simulink model "Orzan_Catalin_Matlab_Simulink"  (R2016a)
settings: Solver=VariableStepAuto  StartTime=0.0  StopTime=10.0  RelTol=1e-3
libraries: mblibv1 x17, simulink_extras x5
settings Model: Creator=Cata  LastModifiedBy=Cata

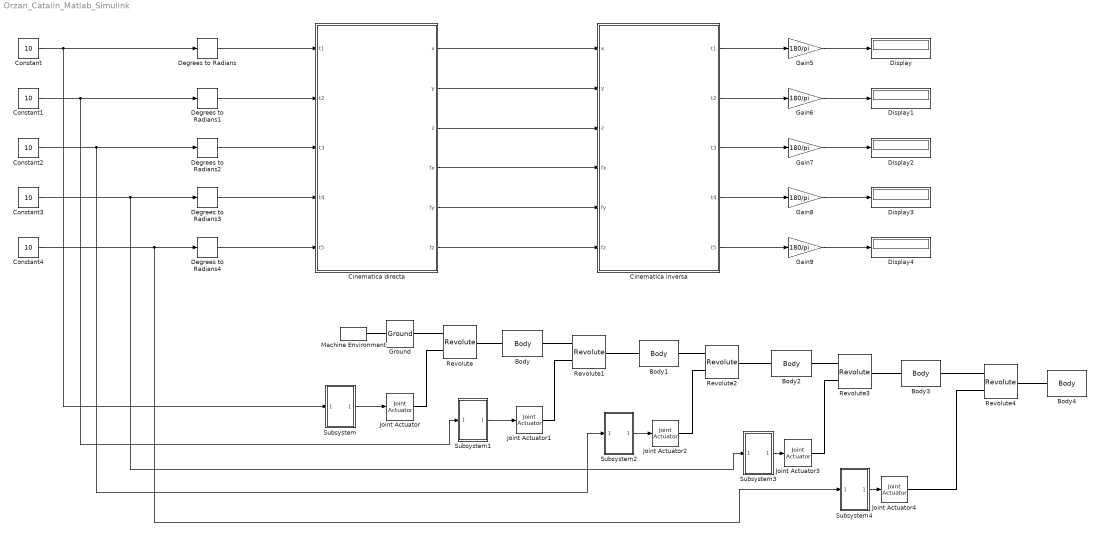
== system Orzan_Catalin_Matlab_Simulink ==
  Body : mblibv1/Bodies/Body  LConnTagsString=CS1  RConnTagsString=CS2  UpdateFromCAD=off  DialogClass=MechanicalBodyBlock  Mass=1  MassUnits=kg  InertiaUnits=kg*m^2  Inertia=eye(3)  Shape=Cylinder  ShapeDims=[1 1]  ShapeUnits=m  ShapeUse=false  Density=1  DensityUnits=kg/m^3  DensityUse=false  GraphicsMode=MACHINE_DEFAULT  BodyColorSelMode=MACHINE_DEFAULT  BodyColor=[1 0 0]  AttachedToCS=CG  CG=Left$CG$[0 0 0]$WORLD$WORLD$mm$[0 0 0]$Euler X-Y-Z$deg$WORLD$false$none  WorkingFrames=Left$CS1$[0 0 0]$World$World$mm$[0 0 0]$Euler X-Y-Z$deg$WORLD$true$none#Right$CS2$[0 0 200]$World$World$mm$[0 0 0]$Euler X-Y-Z$deg$WORLD$true$none  CGPos=[0 0 0]  CGRot=[0 0 0]  CS0Pos=[]  CS0Rot=[]  CS1Pos=[0 0 0]  CS1Rot=[0 0 0]  CS2Pos=[0 0 200]  CS2Rot=[0 0 0]  CS3Pos=[]  CS3Rot=[]  CS4Pos=[]  CS4Rot=[]  CS5Pos=[]  CS5Rot=[]  CS6Pos=[]  CS6Rot=[]  CS7Pos=[]  CS7Rot=[]  CS8Pos=[]  CS8Rot=[]  CS9Pos=[]  CS9Rot=[]  CS10Pos=[]  CS10Rot=[]  CS11Pos=[]  CS11Rot=[]  CS12Pos=[]  CS12Rot=[]  CS13Pos=[]  CS13Rot=[]  CS14Pos=[]  CS14Rot=[]  CS15Pos=[]  CS15Rot=[]  CS16Pos=[]  CS16Rot=[]  CS17Pos=[]  CS17Rot=[]  CS18Pos=[]  CS18Rot=[]  CS19Pos=[]  CS19Rot=[]  CS20Pos=[]  CS20Rot=[]
  Body1 : mblibv1/Bodies/Body  LConnTagsString=CS1  RConnTagsString=CS2  UpdateFromCAD=off  DialogClass=MechanicalBodyBlock  Mass=1  MassUnits=kg  InertiaUnits=kg*m^2  Inertia=eye(3)  Shape=Cylinder  ShapeDims=[1 1]  ShapeUnits=m  ShapeUse=false  Density=1  DensityUnits=kg/m^3  DensityUse=false  GraphicsMode=MACHINE_DEFAULT  BodyColorSelMode=MACHINE_DEFAULT  BodyColor=[1 0 0]  AttachedToCS=CG  CG=Left$CG$[0 0 200]$WORLD$WORLD$mm$[0 0 0]$Euler X-Y-Z$deg$WORLD$false$none  WorkingFrames=Left$CS1$[0 0 200]$World$World$mm$[0 0 0]$Euler X-Y-Z$deg$WORLD$true$none#Right$CS2$[0 0 400]$World$World$mm$[0 0 0]$Euler X-Y-Z$deg$WORLD$true$none  CGPos=[0 0 200]  CGRot=[0 0 0]  CS0Pos=[]  CS0Rot=[]  CS1Pos=[0 0 200]  CS1Rot=[0 0 0]  CS2Pos=[0 0 400]  CS2Rot=[0 0 0]  CS3Pos=[]  CS3Rot=[]  CS4Pos=[]  CS4Rot=[]  CS5Pos=[]  CS5Rot=[]  CS6Pos=[]  CS6Rot=[]  CS7Pos=[]  CS7Rot=[]  CS8Pos=[]  CS8Rot=[]  CS9Pos=[]  CS9Rot=[]  CS10Pos=[]  CS10Rot=[]  CS11Pos=[]  CS11Rot=[]  CS12Pos=[]  CS12Rot=[]  CS13Pos=[]  CS13Rot=[]  CS14Pos=[]  CS14Rot=[]  CS15Pos=[]  CS15Rot=[]  CS16Pos=[]  CS16Rot=[]  CS17Pos=[]  CS17Rot=[]  CS18Pos=[]  CS18Rot=[]  CS19Pos=[]  CS19Rot=[]  CS20Pos=[]  CS20Rot=[]
  Body2 : mblibv1/Bodies/Body  LConnTagsString=CS1  RConnTagsString=CS2  UpdateFromCAD=off  DialogClass=MechanicalBodyBlock  Mass=1  MassUnits=kg  InertiaUnits=kg*m^2  Inertia=eye(3)  Shape=Cylinder  ShapeDims=[1 1]  ShapeUnits=m  ShapeUse=false  Density=1  DensityUnits=kg/m^3  DensityUse=false  GraphicsMode=MACHINE_DEFAULT  BodyColorSelMode=MACHINE_DEFAULT  BodyColor=[1 0 0]  AttachedToCS=CG  CG=Left$CG$[0 0 400]$WORLD$WORLD$mm$[0 0 0]$Euler X-Y-Z$deg$WORLD$false$none  WorkingFrames=Left$CS1$[0 0 400]$World$World$mm$[0 0 0]$Euler X-Y-Z$deg$WORLD$true$none#Right$CS2$[200 0 400]$World$World$mm$[0 0 0]$Euler X-Y-Z$deg$WORLD$true$none  CGPos=[0 0 400]  CGRot=[0 0 0]  CS0Pos=[]  CS0Rot=[]  CS1Pos=[0 0 400]  CS1Rot=[0 0 0]  CS2Pos=[200 0 400]  CS2Rot=[0 0 0]  CS3Pos=[]  CS3Rot=[]  CS4Pos=[]  CS4Rot=[]  CS5Pos=[]  CS5Rot=[]  CS6Pos=[]  CS6Rot=[]  CS7Pos=[]  CS7Rot=[]  CS8Pos=[]  CS8Rot=[]  CS9Pos=[]  CS9Rot=[]  CS10Pos=[]  CS10Rot=[]  CS11Pos=[]  CS11Rot=[]  CS12Pos=[]  CS12Rot=[]  CS13Pos=[]  CS13Rot=[]  CS14Pos=[]  CS14Rot=[]  CS15Pos=[]  CS15Rot=[]  CS16Pos=[]  CS16Rot=[]  CS17Pos=[]  CS17Rot=[]  CS18Pos=[]  CS18Rot=[]  CS19Pos=[]  CS19Rot=[]  CS20Pos=[]  CS20Rot=[]
  Body3 : mblibv1/Bodies/Body  LConnTagsString=CS1  RConnTagsString=CS2  UpdateFromCAD=off  DialogClass=MechanicalBodyBlock  Mass=10  MassUnits=kg  InertiaUnits=kg*m^2  Inertia=eye(3)  Shape=Cylinder  ShapeDims=[1 1]  ShapeUnits=m  ShapeUse=false  Density=1  DensityUnits=kg/m^3  DensityUse=false  GraphicsMode=MACHINE_DEFAULT  BodyColorSelMode=MACHINE_DEFAULT  BodyColor=[1 0 0]  AttachedToCS=CG  CG=Left$CG$[200 0 400]$WORLD$WORLD$mm$[0 0 0]$Euler X-Y-Z$deg$WORLD$false$none  WorkingFrames=Left$CS1$[200 0 400]$World$World$mm$[0 0 0]$Euler X-Y-Z$deg$WORLD$true$none#Right$CS2$[200 0 200]$World$World$mm$[0 0 0]$Euler X-Y-Z$deg$WORLD$true$none  CGPos=[200 0 400]  CGRot=[0 0 0]  CS0Pos=[]  CS0Rot=[]  CS1Pos=[200 0 400]  CS1Rot=[0 0 0]  CS2Pos=[200 0 200]  CS2Rot=[0 0 0]  CS3Pos=[]  CS3Rot=[]  CS4Pos=[]  CS4Rot=[]  CS5Pos=[]  CS5Rot=[]  CS6Pos=[]  CS6Rot=[]  CS7Pos=[]  CS7Rot=[]  CS8Pos=[]  CS8Rot=[]  CS9Pos=[]  CS9Rot=[]  CS10Pos=[]  CS10Rot=[]  CS11Pos=[]  CS11Rot=[]  CS12Pos=[]  CS12Rot=[]  CS13Pos=[]  CS13Rot=[]  CS14Pos=[]  CS14Rot=[]  CS15Pos=[]  CS15Rot=[]  CS16Pos=[]  CS16Rot=[]  CS17Pos=[]  CS17Rot=[]  CS18Pos=[]  CS18Rot=[]  CS19Pos=[]  CS19Rot=[]  CS20Pos=[]  CS20Rot=[]
  Body4 : mblibv1/Bodies/Body  LConnTagsString=CS1  UpdateFromCAD=off  DialogClass=MechanicalBodyBlock  Mass=10  MassUnits=kg  InertiaUnits=kg*m^2  Inertia=eye(3)  Shape=Cylinder  ShapeDims=[1 1]  ShapeUnits=m  ShapeUse=false  Density=1  DensityUnits=kg/m^3  DensityUse=false  GraphicsMode=MACHINE_DEFAULT  BodyColorSelMode=MACHINE_DEFAULT  BodyColor=[1 0 0]  AttachedToCS=CG  CG=Left$CG$[200 0 200]$WORLD$WORLD$mm$[0 0 0]$Euler X-Y-Z$deg$WORLD$false$none  WorkingFrames=Left$CS1$[200 0 200]$World$World$mm$[0 0 0]$Euler X-Y-Z$deg$WORLD$true$none#Right$CS2$[200 0 0]$World$World$mm$[0 0 0]$Euler X-Y-Z$deg$WORLD$false$none  CGPos=[200 0 200]  CGRot=[0 0 0]  CS0Pos=[]  CS0Rot=[]  CS1Pos=[200 0 200]  CS1Rot=[0 0 0]  CS2Pos=[200 0 0]  CS2Rot=[0 0 0]  CS3Pos=[]  CS3Rot=[]  CS4Pos=[]  CS4Rot=[]  CS5Pos=[]  CS5Rot=[]  CS6Pos=[]  CS6Rot=[]  CS7Pos=[]  CS7Rot=[]  CS8Pos=[]  CS8Rot=[]  CS9Pos=[]  CS9Rot=[]  CS10Pos=[]  CS10Rot=[]  CS11Pos=[]  CS11Rot=[]  CS12Pos=[]  CS12Rot=[]  CS13Pos=[]  CS13Rot=[]  CS14Pos=[]  CS14Rot=[]  CS15Pos=[]  CS15Rot=[]  CS16Pos=[]  CS16Rot=[]  CS17Pos=[]  CS17Rot=[]  CS18Pos=[]  CS18Rot=[]  CS19Pos=[]  CS19Rot=[]  CS20Pos=[]  CS20Rot=[]
  "Cinematica directa " : MATLAB Function  TreatAsAtomicUnit=on
  Cinematica inversa : MATLAB Function  TreatAsAtomicUnit=on
  Constant{,1..4} (5 alike) : Constant  Value=10
  Degrees to Radians{,1..4} (5 alike) : simulink_extras/Transformations/Degrees to Radians
  Display{,1..4} (5 alike) : Display
  Gain{5..9} (5 alike) : Gain  Gain=180/pi
  Ground : mblibv1/Bodies/Ground  UpdateFromCAD=off  LeftPortType=env  RightPortType=workingframe  PhysicalDomain=Mechanical  DialogClass=GroundBlock  CoordPosition=[0 0 0]  CoordPositionUnits=m  StateVectorMgrId=0  MachineId=[1 0]  ShowEnvPort=on  ParameterChecksum=[4168860495, 2563258822, 2023213708, 520383932]  TopologyChecksum=[1341745960, 1067854235, 1921025474, 1139980135]
  Joint Actuator{,1..4} (5 alike) : mblibv1/Sensors &  Actuators/Joint Actuator  UpdateFromCAD=off  PhysicalDomain=Mechanical  PortType=blob  ActuationStyle=Motion  AngleUnits=deg  ArcVelocityUnits=deg/s  ArcAccelerationUnits=deg/s^2  CoordPositionUnits=m  VelocityUnits=m/s  AccelerationUnits=m/s^2  ForceUnits=N  TorqueUnits=N*m  ActiveIO=on  Width=3  DialogClass=MechanicalActuatorBlock  Primitive=R1  ReferenceFrame=Absolute (World)
  Machine Environment : mblibv1/Bodies/Machine Environment  PortType=env  PhysicalDomain=Mechanical  DialogTemplateClass=MECH.MachineEnvironment  SyncWhenCopied=off  Gravity=[0 -9.81 0]  GravityUnits=m/s^2  GravityAsSignal=off  Dimensionality=Auto-detect  AnalysisType=Forward dynamics  LinearAssemblyTolerance=1e-3  LinearAssemblyToleranceUnits=m  AngularAssemblyTolerance=1e-3  AngularAssemblyToleranceUnits=rad  ConstraintSolverType=Stabilizing  ConstraintRelTolerance=1e-4  ConstraintAbsTolerance=1e-4  UseRobustSingularityHandling=off  RedundancyAnalysisToleranceType=Automatically select tolerance  RedundancyAnalysisTolerance=1e-14  StatePerturbationType=Fixed  PerturbationSize=1e-5  VisualizeMachine=on  BodyVisualizationType=Use model default body geometries  BodyColorSelMode=Use model default  DefaultBodyColor=[1 0 0]
  Revolute : mblibv1/Joints/Revolute  LConnTagsString=__newl0|SA1  RConnTagsString=__newr0  UpdateFromCAD=off  NumSAPorts=1  CutJoint=off  MarkAsCut=off  Primitives=prismatic  PrimitiveProps=R1$World$[0 0 1]$revolute  DialogClass=JointBlock  R1Axis=[0 0 1]
  Revolute1 : mblibv1/Joints/Revolute  LConnTagsString=__newl0|SA1  RConnTagsString=__newr0  UpdateFromCAD=off  NumSAPorts=1  CutJoint=off  MarkAsCut=off  Primitives=prismatic  PrimitiveProps=R1$World$[0 1 0]$revolute  DialogClass=JointBlock  R1Axis=[0 1 0]
  Revolute2 : mblibv1/Joints/Revolute  LConnTagsString=__newl0|SA1  RConnTagsString=__newr0  UpdateFromCAD=off  NumSAPorts=1  CutJoint=off  MarkAsCut=off  Primitives=prismatic  PrimitiveProps=R1$World$[0 1 0]$revolute  DialogClass=JointBlock  R1Axis=[0 1 0]
  Revolute3 : mblibv1/Joints/Revolute  LConnTagsString=__newl0|SA1  RConnTagsString=__newr0  UpdateFromCAD=off  NumSAPorts=1  CutJoint=off  MarkAsCut=off  Primitives=prismatic  PrimitiveProps=R1$World$[0 1 0]$revolute  DialogClass=JointBlock  R1Axis=[0 1 0]
  Revolute4 : mblibv1/Joints/Revolute  LConnTagsString=__newl0|SA1  RConnTagsString=__newr0  UpdateFromCAD=off  NumSAPorts=1  CutJoint=off  MarkAsCut=off  Primitives=prismatic  PrimitiveProps=R1$World$[1 0 0]$revolute  DialogClass=JointBlock  R1Axis=[1 0 0]
  Subsystem : Subsystem
  Subsystem1 : Subsystem
  Subsystem2 : Subsystem
  Subsystem3 : Subsystem
  Subsystem4 : Subsystem
  wires:
  Constant3/1 -> Subsystem3/1(In1), Degrees to Radians3/1
  Constant2/1 -> Subsystem2/1(In1), Degrees to Radians2/1
  Constant1/1 -> Subsystem1/1(In1), Degrees to Radians1/1
  Constant/1 -> Subsystem/1(In1), Degrees to Radians/1
  Subsystem/1(Out1) -> Joint Actuator/1
  Subsystem1/1(Out1) -> Joint Actuator1/1
  Subsystem2/1(Out1) -> Joint Actuator2/1
  Subsystem3/1(Out1) -> Joint Actuator3/1
  Subsystem4/1(Out1) -> Joint Actuator4/1
  Constant4/1 -> Subsystem4/1(In1), Degrees to Radians4/1
  Cinematica inversa/1(t1) -> Gain5/1
  Cinematica inversa/5(t5) -> Gain9/1
  Cinematica inversa/4(t4) -> Gain8/1
  Cinematica inversa/3(t3) -> Gain7/1
  Cinematica inversa/2(t2) -> Gain6/1
  Gain5/1 -> Display/1
  Gain9/1 -> Display4/1
  Gain8/1 -> Display3/1
  Gain7/1 -> Display2/1
  Gain6/1 -> Display1/1
  "Cinematica directa "/6(fz) -> Cinematica inversa/6(fz)
  "Cinematica directa "/5(fy) -> Cinematica inversa/5(fy)
  "Cinematica directa "/4(fx) -> Cinematica inversa/4(fx)
  "Cinematica directa "/3(z) -> Cinematica inversa/3(z)
  "Cinematica directa "/2(y) -> Cinematica inversa/2(y)
  "Cinematica directa "/1(x) -> Cinematica inversa/1(x)
  Degrees to Radians4/1 -> "Cinematica directa "/5(t5)
  Degrees to Radians3/1 -> "Cinematica directa "/4(t4)
  Degrees to Radians2/1 -> "Cinematica directa "/3(t3)
  Degrees to Radians1/1 -> "Cinematica directa "/2(t2)
  Degrees to Radians/1 -> "Cinematica directa "/1(t1)
  connections:
  Ground/RConn1 -- Revolute/LConn1
  Revolute/RConn1 -- Body/LConn1
  Body/RConn1 -- Revolute1/LConn1
  Revolute1/RConn1 -- Body1/LConn1
  Body1/RConn1 -- Revolute2/LConn1
  Revolute2/RConn1 -- Body2/LConn1
  Body2/RConn1 -- Revolute3/LConn1
  Revolute3/RConn1 -- Body3/LConn1
  Joint Actuator/RConn1 -- Revolute/LConn2
  Joint Actuator1/RConn1 -- Revolute1/LConn2
  Joint Actuator2/RConn1 -- Revolute2/LConn2
  Joint Actuator3/RConn1 -- Revolute3/LConn2
  Machine Environment/RConn1 -- Ground/LConn1
  Revolute4/RConn1 -- Body4/LConn1
  Revolute4/LConn1 -- Body3/RConn1
  Revolute4/LConn2 -- Joint Actuator4/RConn1

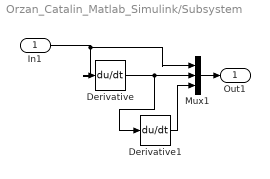
== system Orzan_Catalin_Matlab_Simulink/Subsystem ==
  In1 : Inport
  Derivative : Derivative
  Derivative1 : Derivative
  Mux1 : Mux  Inputs=3
  Out1 : Outport
  wires:
  Derivative/1 -> Derivative1/1, Mux1/2
  Mux1/1 -> Out1/1
  In1/1 -> Derivative/1, Mux1/1
  Derivative1/1 -> Mux1/3

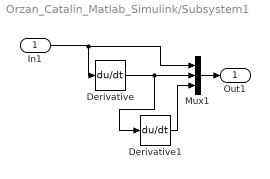
== system Orzan_Catalin_Matlab_Simulink/Subsystem1 ==
  In1 : Inport
  Derivative : Derivative
  Derivative1 : Derivative
  Mux1 : Mux  Inputs=3
  Out1 : Outport
  wires:
  Derivative/1 -> Derivative1/1, Mux1/2
  Mux1/1 -> Out1/1
  In1/1 -> Derivative/1, Mux1/1
  Derivative1/1 -> Mux1/3

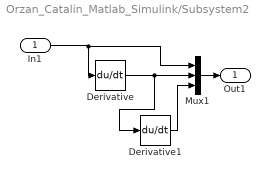
== system Orzan_Catalin_Matlab_Simulink/Subsystem2 ==
  In1 : Inport
  Derivative : Derivative
  Derivative1 : Derivative
  Mux1 : Mux  Inputs=3
  Out1 : Outport
  wires:
  Derivative/1 -> Derivative1/1, Mux1/2
  Mux1/1 -> Out1/1
  In1/1 -> Derivative/1, Mux1/1
  Derivative1/1 -> Mux1/3

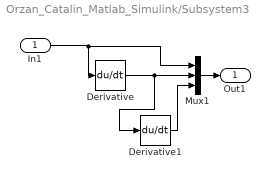
== system Orzan_Catalin_Matlab_Simulink/Subsystem3 ==
  In1 : Inport
  Derivative : Derivative
  Derivative1 : Derivative
  Mux1 : Mux  Inputs=3
  Out1 : Outport
  wires:
  Derivative/1 -> Derivative1/1, Mux1/2
  Mux1/1 -> Out1/1
  In1/1 -> Derivative/1, Mux1/1
  Derivative1/1 -> Mux1/3

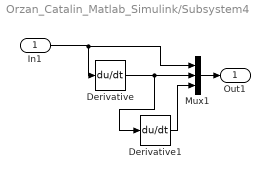
== system Orzan_Catalin_Matlab_Simulink/Subsystem4 ==
  In1 : Inport
  Derivative : Derivative
  Derivative1 : Derivative
  Mux1 : Mux  Inputs=3
  Out1 : Outport
  wires:
  Derivative/1 -> Derivative1/1, Mux1/2
  Mux1/1 -> Out1/1
  In1/1 -> Derivative/1, Mux1/1
  Derivative1/1 -> Mux1/3

== matlab function Orzan_Catalin_Matlab_Simulink/Cinematica inversa ==
  data: t1 output; x input; t2 output; y input; z input; fx input; fy input; t3 output; t4 output; t5 output; fz input

function [t1, t2, t3, t4, t5]= fcn(x, y, z, fx, fy, fz)

Tx=[1 0 0 x; 0 1 0 0; 0 0 1 0; 0 0 0 1];
Ty=[1 0 0 0; 0 1 0 y; 0 0 1 0; 0 0 0 1];
Tz=[1 0 0 0; 0 1 0 0; 0 0 1 z; 0 0 0 1];

Rx=[1 0 0 0; 0 cos(fx) -sin(fx) 0; 0 sin(fx) cos(fx) 0; 0 0 0 1];
Ry=[cos(fy) 0 sin(fy) 0; 0 1 0 0; -sin(fy) 0 cos(fy) 0; 0 0 0 1];
Rz=[cos(fz) -sin(fz) 0 0; sin(fz) cos(fz) 0 0; 0 0 1 0; 0 0 0 1];

H=Tx*Ty*Tz*Rz*Ry*Rx;

A9=[1 0 0 0; 0 1 0 0; 0 0 1 -200; 0 0 0 1];

Hc=H*A9^(-1);

xc=Hc(1,4);
yc=Hc(2,4);
zc=Hc(3,4);

t1=atan(yc/xc);
 
A1=[cos(t1) -sin(t1) 0 0; sin(t1) cos(t1) 0 0; 0 0 1 0; 0 0 0 1];
A2=[1 0 0 0; 0 1 0 0; 0 0 1 200; 0 0 0 1];

Ha=A1*A2;

xa=Ha(1,4);
ya=Ha(2,4);
za=Ha(3,4);

L0=sqrt((xc-xa)^2+(yc-ya)^2+(zc-za)^2);
L1=sqrt((xc)^2+(yc)^2);
L2=sqrt((L0)^2-(L1)^2);
alpha=acos((L0^2-200^2-200^2)/(2*200*200));

t3=alpha-(pi/2);

beta=atan(L2/L1);
gama=acos((200^2-200^2-L0^2)/(2*200*L0));
t2=-((beta-gama)+pi/2);

A3 = [cos(t2) 0 sin(t2) 0; 0 1 0 0; -sin(t2), 0, cos(t2), 0; 0 0 0 1];
A4=[1 0 0 0; 0 1 0 0; 0 0 1 200; 0 0 0 1];
A5=[cos(t3) 0 sin(t3) 0; 0 1 0 0; -sin(t3) 0 cos(t3) 0; 0 0 0 1];
A6=[1 0 0 200; 0 1 0 0; 0 0 1 0; 0 0 0 1];

H1=A1*A2*A3*A4*A5*A6;
H2=H1^(-1)*H*A9^(-1);

t4=-atan(H2(3,1)/H2(1,1));
t5=-atan(H2(2,3)/H2(2,2));

== matlab function Orzan_Catalin_Matlab_Simulink/Cinematica directa  ==
  data: x output; t1 input; y output; t2 input; t3 input; t4 input; t5 input; z output; fx output; fy output; fz output

function [x, y, z, fx, fy, fz]= fcn(t1, t2, t3, t4, t5)

A1=[cos(t1) -sin(t1) 0 0; sin(t1) cos(t1) 0 0; 0 0 1 0; 0 0 0 1];
A2=[1 0 0 0; 0 1 0 0; 0 0 1 200; 0 0 0 1];
A3 = [cos(t2) 0 sin(t2) 0; 0 1 0 0; -sin(t2), 0, cos(t2), 0; 0 0 0 1];
A4=[1 0 0 0; 0 1 0 0; 0 0 1 200; 0 0 0 1];
A5=[cos(t3) 0 sin(t3) 0; 0 1 0 0; -sin(t3) 0 cos(t3) 0; 0 0 0 1];
A6=[1 0 0 200; 0 1 0 0; 0 0 1 0; 0 0 0 1];
A7=[cos(t4) 0 sin(t4) 0; 0 1 0 0; -sin(t4) 0 cos(t4) 0; 0 0 0 1];
A8=[1 0 0 0; 0 cos(t5) -sin(t5) 0; 0 sin(t5) cos(t5) 0; 0 0 0 1];
A9=[1 0 0 0; 0 1 0 0; 0 0 1 -200; 0 0 0 1];



H=A1*A2*A3*A4*A5*A6*A7*A8*A9;
x=H(1,4);
y=H(2,4);
z=H(3,4);
fx=atan2(H(3,2),H(3,3));
fy=-asin(H(3,1));
fz=atan2(H(2,1),H(1,1));
